simulink model "QPSK_task_3"  (R2018a)
settings: Solver=VariableStepAuto  StartTime=0.0  StopTime=10  RelTol=1e-3
libraries: commdigbbndpm3 x2, commchan3 x1, commrandsrc3 x1, commsink2 x1
settings Model: Creator=Sheikh  LastModifiedBy=Sheikh

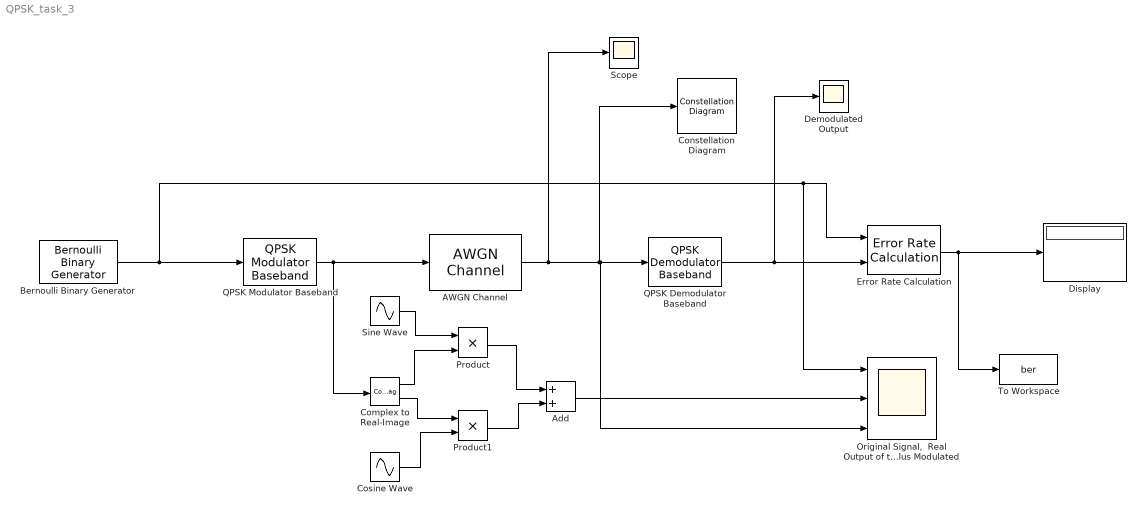
== system QPSK_task_3 ==
  AWGN Channel : commchan3/AWGN Channel  InputProcessing=Columns as channels (frame based)  seed=67  noiseMode="Signal to noise ratio  (Eb/No)"  EbNodB=10  EsNodB=10  SNRdB=10  bitsPerSym=2  Ps=1  Tsym=1  variance=1
  Add : Sum
  Bernoulli Binary Generator : commrandsrc3/Bernoulli Binary Generator  ProbabilityOfZero=0.5  SeedSource=Parameter  Seed=37  SampleTime=0.1  SamplesPerFrame=1  OutputDataType=double  SimulateUsing=Interpreted execution
  Complex to Real-Image : ComplexToRealImag
  Constellation Diagram : ConstellationDiagram
  "Cosine Wave " : Sin  Frequency=2*pi*4  Phase=pi/2  SampleTime=0.01
  Demodulated Output : Scope
  Display : Display
  Error Rate Calculation : commsink2/Error Rate Calculation  N=0  st_delay=0  cp_mode=Entire frame  subframe=[]  PMode=Port  WsName=ErrorVec  RsMode2=off  stop=on  numErr=1000  maxBits=1e16
  "Original Signal,  Real Output of the Modulator, Noise Plus Modulated" : Scope  NumInputPorts=3
  Product : Product
  Product1 : Product
  QPSK Demodulator Baseband : commdigbbndpm3/QPSK Demodulator Baseband  OutType=Integer  DecType=Hard decision  VarSource=Dialog  Variance=1  Dec=Gray  Ph=pi/4  outDtype1=Inherit via internal rule  outDtype2=Inherit via internal rule  derotateFactorWordLen=16  derotateFactorDataTypeStr=Inherit: Same word length as input  derotateFactorLastDataTypeStr=Inherit: Same word length as input
  QPSK Modulator Baseband : commdigbbndpm3/QPSK Modulator Baseband  InType=Integer  Enc=Gray  Ph=pi/4  outDtype=double  outWordLen=16  outUDDataType=sfix(16)  outFracLenMode=Best precision  outFracLen=15  outDataTypeStr=double  outLastDataTypeStr=double
  Scope : Scope
  Sine Wave : Sin  Frequency=2*pi*4  SampleTime=0.01
  To Workspace : ToWorkspace  VariableName=ber  SampleTime=-1
      settings: MaxDataPoints=2  Save2DSignal=2-D array (concatenate along first dimension)
  wires:
  Add/1 -> "Original Signal,  Real Output of the Modulator, Noise Plus Modulated"/2
  Error Rate Calculation/1 -> To Workspace/1, Display/1
  "Cosine Wave "/1 -> Product1/2
  Sine Wave/1 -> Product/1
  QPSK Modulator Baseband/1 -> Complex to Real-Image/1, AWGN Channel/1
  Product/1 -> Add/1
  AWGN Channel/1 -> Scope/1, QPSK Demodulator Baseband/1, "Original Signal,  Real Output of the Modulator, Noise Plus Modulated"/3, Constellation Diagram/1
  Complex to Real-Image/2 -> Product1/1
  QPSK Demodulator Baseband/1 -> Demodulated Output/1, Error Rate Calculation/2
  Product1/1 -> Add/2
  Complex to Real-Image/1 -> Product/2
  Bernoulli Binary Generator/1 -> QPSK Modulator Baseband/1, "Original Signal,  Real Output of the Modulator, Noise Plus Modulated"/1, Error Rate Calculation/1
